simulink model "SuspensionModel"  (R2021a)
settings: Solver=VariableStepAuto  StartTime=0.0  StopTime=10.0  RelTol=1e-3
values from neighbouring files (symbols this model uses):
  k = [105.94; 145.76]    [suspensiontest.m]
  l = [531.71; 104.46]    [suspensiontest.m]
  x = linspace(pi, 2 * pi, 50000)    [Camber_WheelTravel.m]    (also in suspensiontest.m = [245; 307.03])
  y = [245; 393.73]    [suspensiontest.m]
  z = -xc*cos(th0rest)-yc*sin(th0rest)    [refactoredcamberrate.m]    (also in suspensiontest.m = [105.94; 145.76])
settings Model: Creator=mreyn  LastModifiedBy=n10234586

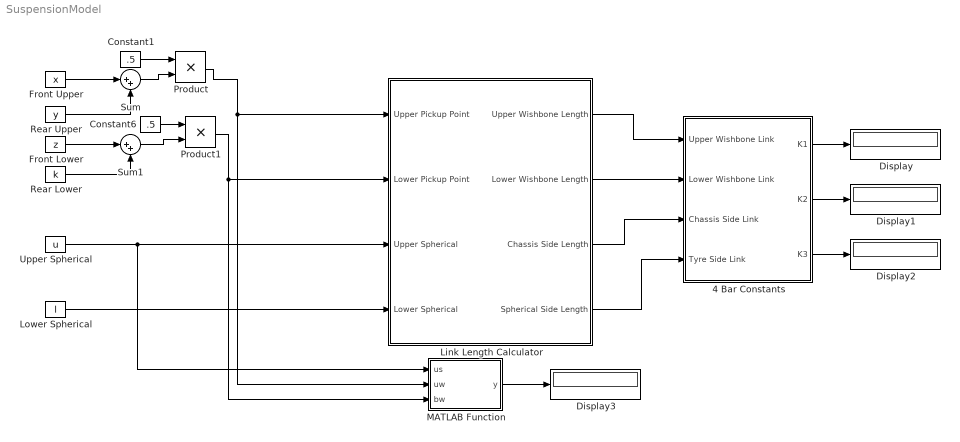
== system SuspensionModel ==
  4 Bar Constants : Subsystem
  Constant1 : Constant  Value=.5
  Constant6 : Constant  Value=.5
  Display{,1..3} (4 alike) : Display
  Front Lower : Constant  Value=z
  Front Upper : Constant  Value=x
  Link Length Calculator : Subsystem
  Lower Spherical : Constant  Value=l
  MATLAB Function : MATLAB Function  TreatAsAtomicUnit=on
  Product : Product
  Product1 : Product
  Rear Lower : Constant  Value=k
  Rear Upper : Constant  Value=y
  Sum : Sum  Inputs=|++
  Sum1 : Sum  Inputs=|++
  Upper Spherical : Constant  Value=u
  wires:
  Front Lower/1 -> Sum1/1
  Rear Upper/1 -> Sum/2
  Front Upper/1 -> Sum/1
  Rear Lower/1 -> Sum1/2
  Constant1/1 -> Product/1
  Sum/1 -> Product/2
  Product/1 -> MATLAB Function/2(uw), Link Length Calculator/1(Upper Pickup Point)
  Constant6/1 -> Product1/1
  Sum1/1 -> Product1/2
  Product1/1 -> MATLAB Function/3(bw), Link Length Calculator/2(Lower Pickup Point)
  Upper Spherical/1 -> MATLAB Function/1(us), Link Length Calculator/3(Upper Spherical)
  Lower Spherical/1 -> Link Length Calculator/4(Lower Spherical)
  Link Length Calculator/1(Upper Wishbone Length) -> 4 Bar Constants/1(Upper Wishbone Link)
  Link Length Calculator/2(Lower Wishbone Length) -> 4 Bar Constants/2(Lower Wishbone Link)
  Link Length Calculator/3(Chassis Side Length) -> 4 Bar Constants/3(Chassis Side Link)
  Link Length Calculator/4(Spherical Side Length) -> 4 Bar Constants/4(Tyre Side Link)
  4 Bar Constants/1(K1) -> Display/1
  4 Bar Constants/2(K2) -> Display1/1
  4 Bar Constants/3(K3) -> Display2/1
  MATLAB Function/1(y) -> Display3/1

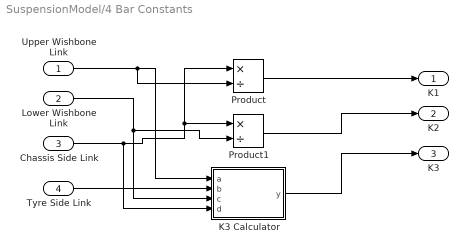
== system SuspensionModel/4 Bar Constants ==
  Upper Wishbone Link : Inport
  Lower Wishbone Link : Inport  Port=2
  Chassis Side Link : Inport  Port=3
  Tyre Side Link : Inport  Port=4
  K3 Calculator : MATLAB Function  TreatAsAtomicUnit=on
  Product : Product  Inputs=*/
  Product1 : Product  Inputs=*/
  K1 : Outport
  K2 : Outport  Port=2
  K3 : Outport  Port=3
  wires:
  Chassis Side Link/1 -> K3 Calculator/4(d), Product1/1, Product/1
  Upper Wishbone Link/1 -> Product/2, K3 Calculator/1(a)
  Product/1 -> K1/1
  Lower Wishbone Link/1 -> Product1/2, K3 Calculator/3(c)
  Product1/1 -> K2/1
  K3 Calculator/1(y) -> K3/1
  Tyre Side Link/1 -> K3 Calculator/2(b)

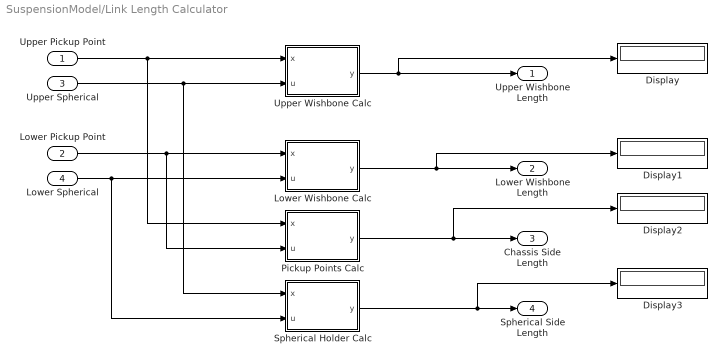
== system SuspensionModel/Link Length Calculator ==
  Upper Pickup Point : Inport
  Lower Pickup Point : Inport  Port=2
  Upper Spherical : Inport  Port=3
  Lower Spherical : Inport  Port=4
  Display{,1..3} (4 alike) : Display
  Lower Wishbone Calc : MATLAB Function  TreatAsAtomicUnit=on
  Pickup Points Calc : MATLAB Function  TreatAsAtomicUnit=on
  Spherical Holder Calc : MATLAB Function  TreatAsAtomicUnit=on
  Upper Wishbone Calc : MATLAB Function  TreatAsAtomicUnit=on
  Upper Wishbone Length : Outport
  Lower Wishbone Length : Outport  Port=2
  Chassis Side Length : Outport  Port=3
  Spherical Side Length : Outport  Port=4
  wires:
  Upper Pickup Point/1 -> Pickup Points Calc/1(x), Upper Wishbone Calc/1(x)
  Upper Spherical/1 -> Spherical Holder Calc/1(x), Upper Wishbone Calc/2(u)
  Lower Pickup Point/1 -> Pickup Points Calc/2(u), Lower Wishbone Calc/1(x)
  Lower Spherical/1 -> Spherical Holder Calc/2(u), Lower Wishbone Calc/2(u)
  Spherical Holder Calc/1(y) -> Display3/1, Spherical Side Length/1
  Pickup Points Calc/1(y) -> Display2/1, Chassis Side Length/1
  Lower Wishbone Calc/1(y) -> Display1/1, Lower Wishbone Length/1
  Upper Wishbone Calc/1(y) -> Display/1, Upper Wishbone Length/1

== matlab function SuspensionModel/Link Length Calculator/Lower Wishbone Calc ==
  data: x input; u input; y output
function y = fcn(x, u)

y = norm(u-x);

== matlab function SuspensionModel/Link Length Calculator/Upper Wishbone Calc ==
  data: x input; u input; y output
function y = fcn(x, u)

y = norm(u-x);

== matlab function SuspensionModel/Link Length Calculator/Pickup Points Calc ==
  data: x input; u input; y output
function y = fcn(x, u)

y = norm(u-x);

== matlab function SuspensionModel/Link Length Calculator/Spherical Holder Calc ==
  data: x input; u input; y output
function y = fcn(x, u)

y = norm(u-x);

== matlab function SuspensionModel/MATLAB Function ==
  data: us input; y output; uw input; bw input
function y = fcn(us, uw, bw)

y = atan((us(2)-uw(2))/abs(us(1)-uw(1)))+(pi/2)+abs(atan((uw(1)-bw(1))/(uw(2)-bw(2))));

== matlab function SuspensionModel/4 Bar Constants/K3 Calculator ==
  data: a input; y output; b input; c input; d input
function y = fcn(a, b, c, d)

y = (a^2+c^2+d^2-b^2)/(2*a*c);
